simulink model "quadcopter_swarm"  (R2023b)
settings: Solver=ode3  StartTime=0  StopTime=50  FixedStep=0.005  RelTol=1e-3  EnableMultiTasking=on
values from neighbouring files (symbols this model uses):
  F_e_g = [0 0 39.28]    [1nrx_dot.mat]    (also in 1nrxdrones_dot.mat; collision_avoidance_POS.mat; collision_avoidance_headonfix_POS.mat; collision_test.mat)
  g = 9.82    [1nrx_dot.mat]    (also in 1nrxdrones_dot.mat; collision_avoidance_POS.mat; collision_avoidance_headonfix_POS.mat; collision_test.mat)
  I_C = [0.5  0  0; 0  0.5  0; 0  0  1]    [1nrx_dot.mat]    (also in 1nrxdrones_dot.mat; collision_avoidance_POS.mat; collision_avoidance_headonfix_POS.mat; collision_test.mat)
  m = 4    [1nrx_dot.mat]    (also in 1nrxdrones_dot.mat; collision_avoidance_POS.mat; collision_avoidance_headonfix_POS.mat; collision_test.mat)
  M_RB = [4 0 0 0 0 0 0 4 0 0 0 0 ... (36 elements, 6x6)]    [1nrx_dot.mat]    (also in 1nrxdrones_dot.mat; collision_avoidance_POS.mat; collision_avoidance_headonfix_POS.mat; collision_test.mat)
undefined symbols (not defined in the file or in its folder): PID_inner_max, PID_outer_max
libraries: slpidlib x24, simulink_extras x20, dspsigops x12, aerolibutil x8, sharedtransform x4, vrlib x1
(part 5 of 5)

== matlab function quadcopter_swarm/Slave drone 3/Quadcopter model Euler/rigid-body dynamics/MATLAB Function ==
  data: tau input; nu_dot output; nu input; I_C input; M_RB input; m input
function nu_dot = fcn(tau,nu,I_C,M_RB,m)

omega_b_b_e = nu(4:6);

C_RB = [
    m*skew_sym(omega_b_b_e)     zeros(3)
    zeros(3)                    -skew_sym(I_C*omega_b_b_e)
];

nu_dot = inv(M_RB)*(tau - C_RB*nu);

end


function res = skew_sym(vector)

res = [
    0               -vector(3)      vector(2)
    vector(3)       0               -vector(1)
    -vector(2)     vector(1)       0
];

end

== matlab function quadcopter_swarm/Master drone/PID controllers/outer-loop position controller/MATLAB Function1 ==
  data: Deltap_e input; Deltap_b output; psi input
function Deltap_b = fcn(Deltap_e,psi)

R = [ cos(psi) , -sin(psi) ;
      sin(psi) ,  cos(psi) ];

Deltap_b = R'*Deltap_e;
